simulink model "controllerCoreAlgorithm"  (R2022a)
settings: configuration reference "ControllerCodeGenerationConfigurationSet" (kept outside this file)
model workspace (MATLAB code in the model file + MAT data in the model file):
  cmdLim = Simulink.Parameter
  cmdLim.Value = 15
  cmdLim.Description = 'Limit for controlling the maximum surface command angle.'
  cmdLim.Min = 0
  cmdLim.Max = 90
  cmdLim.DocUnits = 'deg'
  dispGain = Simulink.Parameter
  dispGain.Value = 0.75
  dispGain.Description = 'Gain applied to the displacement error.'
  dispGain.Min = 0
  dispGain.Max = []
  dispGain.DocUnits = 'deg/sec/deg'
  dispLim = Simulink.Parameter
  dispLim.Value = 30
  dispLim.Description = 'Limit for controlling the maximum commanded angle.'
  dispLim.Min = 0
  dispLim.Max = 180
  dispLim.DocUnits = 'deg'
  intGain = Simulink.Parameter
  intGain.Value = 0.5
  intGain.Description = 'Gain applied to the integral error.'
  intGain.Min = 0
  intGain.Max = []
  intGain.DocUnits = 'deg/sec/deg/sec'
  intLim = Simulink.Parameter
  intLim.Value = 5
  intLim.Description = 'Limit for controlling the maximum commanded angle.'
  intLim.Min = 0
  intLim.Max = 90
  intLim.DocUnits = 'deg'
  rateGain = Simulink.Parameter
  rateGain.Value = 2
  rateGain.Description = 'Gain applied to the rate error.'
  rateGain.Min = 0
  rateGain.Max = []
  rateGain.DocUnits = 'deg/deg/sec'
  rateLim = Simulink.Parameter
  rateLim.Value = 6
  rateLim.Description = 'Limit for controlling the maximum commanded angle.'
  rateLim.Min = 0
  rateLim.Max = 180
  rateLim.DocUnits = 'deg/sec'
  hdgGain = Simulink.Parameter
  hdgGain.Value = 0.015
  CLIENT_DEVICE_ID_LIST = Simulink.Parameter
  CLIENT_DEVICE_ID_LIST.Value(1).device_id = [0; 0; 0; 0; 0; 0; 0; 0; 0; 0]
  CLIENT_DEVICE_ID_LIST.Value(2).device_id = [0; 0; 0; 0; 0; 0; 0; 0; 0; 0]
  CLIENT_DEVICE_ID_LIST.Value(3).device_id = [0; 0; 0; 0; 0; 0; 0; 0; 0; 0]
  CLIENT_DEVICE_ID_LIST.Value(4).device_id = [0; 0; 0; 0; 0; 0; 0; 0; 0; 0]
  CLIENT_DEVICE_ID_LIST.Description = 'repmat( SensorTargetSpecificCodeExternalDependency.deviceIDBusTypeDefaultConstructor( ), 4, 1 )'
  CLIENT_DEVICE_ID_LIST.DataType = 'Bus: DeviceIDBusType'
  CLIENT_DEVICE_ID_LIST.Complexity = 'real'
  CLIENT_DEVICE_ID_LIST.Dimensions = [4 1]
  CONTROLLER_SAMPLE_TIME = 0.01
  RECEPTION_LOSS_MESSAGE_INTERVAL = 2
  TIRE_PRESSURE_LOWER_THRESHOLD = 1.4
  TIRE_PRESSURE_UPPER_THRESHOLD = 4.6
undefined symbols (not defined in the file): DEFAULT_DEVICE_ID, DEFAULT_MEASUREMENT_MSG_BUS_TYPE, deviceID, faultCode, FaultCodeEnumType, logFault, PER_STEP_MAXIMUM_MESSAGES_TO_PROCESS
settings Model: RequirementInfo={} %GIDa_fe9045fd_0412_4b6e_8206_617cc20e6fde  DataDictionary=controllerCoreAlgorithmData.sldd  FPTRunName=Active  ParameterArgumentNames=CLIENT_DEVICE_ID_LIST  Creator=The MathWorks, Inc.  LastModifiedBy=The MathWorks, Inc.
settings ConfigSetRef: SourceName=ControllerCodeGenerationConfigurationSet

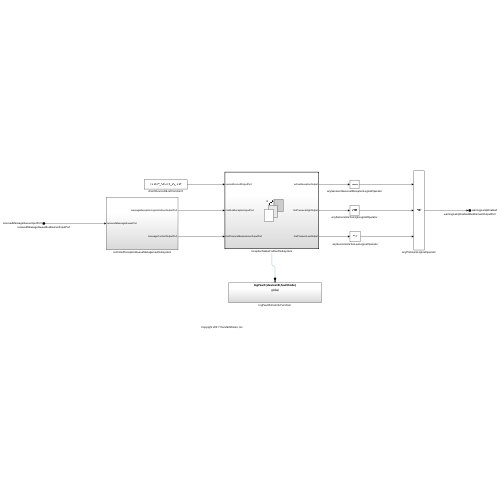
[thumbnail: Simulink's stored preview of the top-level diagram]
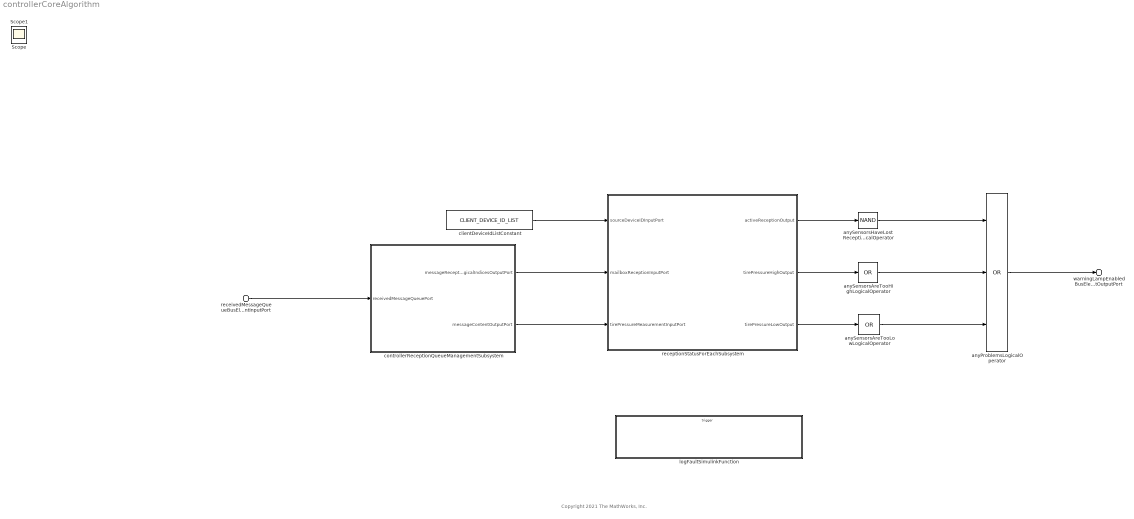
== system controllerCoreAlgorithm ==
  note: Copyright 2021 The MathWorks, Inc.
  receivedMessageQueueBusElementInputPort : Inport  PortName=receivedMessageQueueInputPort
  anyProblemsLogicalOperator : Logic  Operator=OR  Inputs=3  AllPortsSameDT=off  OutDataTypeStr=boolean
  anySensorsAreTooHighLogicalOperator : Logic  Operator=OR  Inputs=1  AllPortsSameDT=off  OutDataTypeStr=boolean
  anySensorsAreTooLowLogicalOperator : Logic  Operator=OR  Inputs=1  AllPortsSameDT=off  OutDataTypeStr=boolean
  anySensorsHaveLostReceptionLogicalOperator : Logic  Operator=NAND  Inputs=1  AllPortsSameDT=off  OutDataTypeStr=boolean
  clientDeviceIdListConstant : Constant  Value=CLIENT_DEVICE_ID_LIST  VectorParams1D=off  OutDataTypeStr=Bus: DeviceIDBusType
  controllerReceptionQueueManagementSubsystem : Subsystem
  logFaultSimulinkFunction : Subsystem  TreatAsAtomicUnit=on
  receptionStatusForEachSubsystem : Subsystem  TreatAsAtomicUnit=on
  warningLampEnabledBusElementOutputPort : Outport  PortName=warningLampEnabled
  Scope : Scope
  Scope1 : Scope
  wires:
  controllerReceptionQueueManagementSubsystem/1(messageReceptionLogicalIndicesOutputPort) -> receptionStatusForEachSubsystem/2(mailboxReceptionInputPort)
  clientDeviceIdListConstant/1 -> receptionStatusForEachSubsystem/1(sourceDeviceIDInputPort)
  receptionStatusForEachSubsystem/1(activeReceptionOutput) -> anySensorsHaveLostReceptionLogicalOperator/1
  receptionStatusForEachSubsystem/2(tirePressureHighOutput) -> anySensorsAreTooHighLogicalOperator/1
  receptionStatusForEachSubsystem/3(tirePressureLowOutput) -> anySensorsAreTooLowLogicalOperator/1
  anySensorsHaveLostReceptionLogicalOperator/1 -> anyProblemsLogicalOperator/1
  anyProblemsLogicalOperator/1 -> warningLampEnabledBusElementOutputPort/1
  anySensorsAreTooHighLogicalOperator/1 -> anyProblemsLogicalOperator/2
  anySensorsAreTooLowLogicalOperator/1 -> anyProblemsLogicalOperator/3
  controllerReceptionQueueManagementSubsystem/2(messageContentOutputPort) -> receptionStatusForEachSubsystem/3(tirePressureMeasurementInputPort)
  receivedMessageQueueBusElementInputPort/1 -> controllerReceptionQueueManagementSubsystem/1(receivedMessageQueuePort)

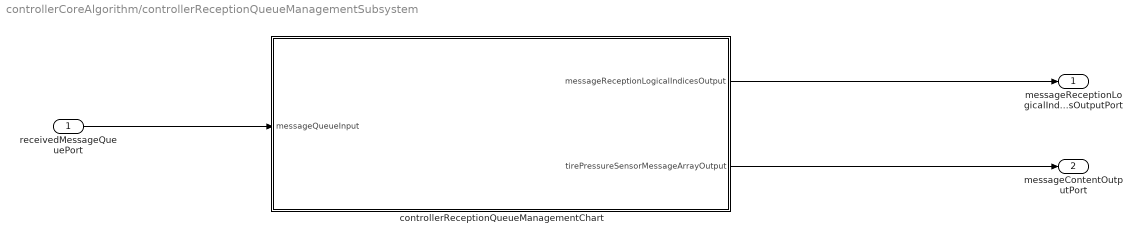
== system controllerCoreAlgorithm/controllerReceptionQueueManagementSubsystem ==
  receivedMessageQueuePort : Inport
  controllerReceptionQueueManagementChart : Stateflow chart  TreatAsAtomicUnit=on
  messageReceptionLogicalIndicesOutputPort : Outport
  messageContentOutputPort : Outport  Port=2
  wires:
  receivedMessageQueuePort/1 -> controllerReceptionQueueManagementChart/1(messageQueueInput)
  controllerReceptionQueueManagementChart/2(tirePressureSensorMessageArrayOutput) -> messageContentOutputPort/1
  controllerReceptionQueueManagementChart/1(messageReceptionLogicalIndicesOutput) -> messageReceptionLogicalIndicesOutputPort/1

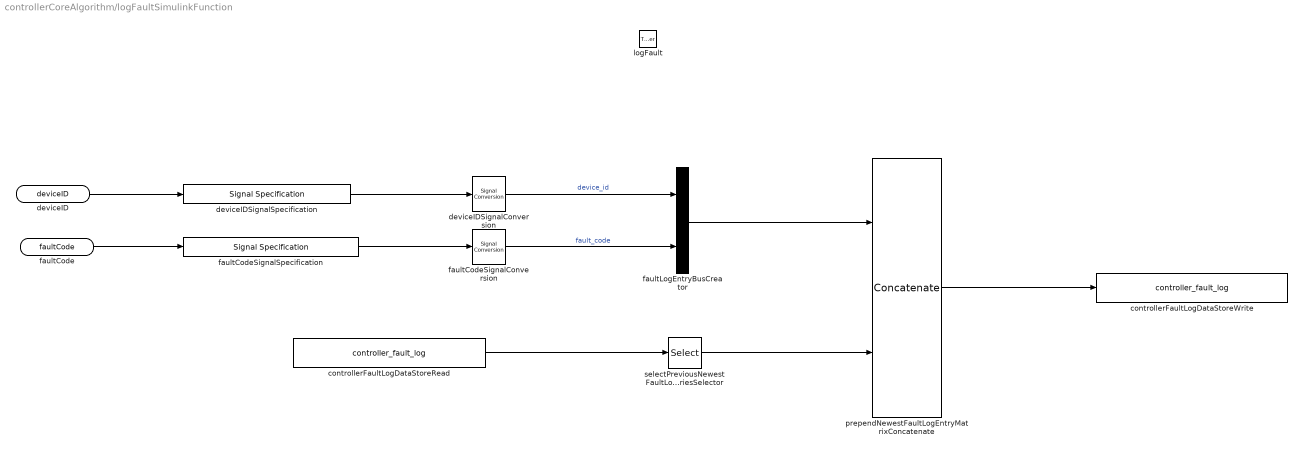
== system controllerCoreAlgorithm/logFaultSimulinkFunction ==
  logFault : TriggerPort  TriggerType=function-call  IsSimulinkFunction=on  FunctionName=logFault  VariantControl=(inherit)
  controllerFaultLogDataStoreRead : DataStoreRead  DataStoreName=controller_fault_log  IndexOptions=Index vector (dialog)  Indices=1  OutputSizes=1
  controllerFaultLogDataStoreWrite : DataStoreWrite  DataStoreName=controller_fault_log  IndexOptions=Index vector (dialog)  Indices=1  OutputSizes=1
  deviceIDSignalConversion : SignalConversion  OverrideOpt=off
  deviceIDSignalSpecification : SignalSpecification  OutDataTypeStr=Bus: DeviceIDBusType  BusOutputAsStruct=on
  faultCodeSignalConversion : SignalConversion  OverrideOpt=off
  faultCodeSignalSpecification : SignalSpecification  OutDataTypeStr=Enum: FaultCodeEnumType
  faultLogEntryBusCreator : BusCreator  Inputs=2  OutDataTypeStr=Bus: ControllerFaultLogEntryBusType  NonVirtualBus=on
  prependNewestFaultLogEntryMatrixConcatenate : Concatenate  Mode=Multidimensional array
  selectPreviousNewestFaultLogEntriesSelector : Selector  InputPortWidth=10  IndexOptions=Index vector (dialog)  Indices=[1: 9]  OutputSizes=1
  deviceID : ArgIn  DisableCoverage=on  OutDataTypeStr=Bus: DeviceIDBusType  ArgumentName=deviceID
  faultCode : ArgIn  DisableCoverage=on  Port=2  OutDataTypeStr=Enum: FaultCodeEnumType  ArgumentName=faultCode
  wires:
  deviceID/1 -> deviceIDSignalSpecification/1
  faultCode/1 -> faultCodeSignalSpecification/1
  deviceIDSignalSpecification/1 -> deviceIDSignalConversion/1
  faultCodeSignalSpecification/1 -> faultCodeSignalConversion/1
  controllerFaultLogDataStoreRead/1 -> selectPreviousNewestFaultLogEntriesSelector/1
  prependNewestFaultLogEntryMatrixConcatenate/1 -> controllerFaultLogDataStoreWrite/1
  faultCodeSignalConversion/1 -> faultLogEntryBusCreator/2  "fault_code"
  deviceIDSignalConversion/1 -> faultLogEntryBusCreator/1  "device_id"
  faultLogEntryBusCreator/1 -> prependNewestFaultLogEntryMatrixConcatenate/1
  selectPreviousNewestFaultLogEntriesSelector/1 -> prependNewestFaultLogEntryMatrixConcatenate/2

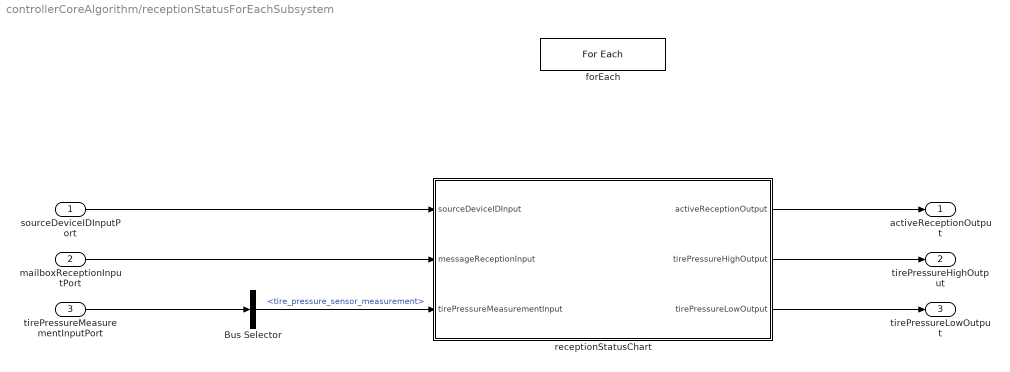
== system controllerCoreAlgorithm/receptionStatusForEachSubsystem ==
  sourceDeviceIDInputPort : Inport  Partition=on  PartitionDimension=1  PartitionWidth=1  PartitionOffset=0
  mailboxReceptionInputPort : Inport  Port=2  Partition=on  PartitionDimension=1  PartitionWidth=1  PartitionOffset=0
  tirePressureMeasurementInputPort : Inport  Port=3  Partition=on  PartitionDimension=1  PartitionWidth=1  PartitionOffset=0
  Bus Selector : BusSelector  OutputSignals=tire_pressure_sensor_measurement
  forEach : ForEach  DisableCoverage=on
  receptionStatusChart : Stateflow chart  TreatAsAtomicUnit=on
      settings: RTWSystemCode=Inline
  activeReceptionOutput : Outport  ConcatenationDimension=1
  tirePressureHighOutput : Outport  Port=2  ConcatenationDimension=1
  tirePressureLowOutput : Outport  Port=3  ConcatenationDimension=1
  wires:
  mailboxReceptionInputPort/1 -> receptionStatusChart/2(messageReceptionInput)
  sourceDeviceIDInputPort/1 -> receptionStatusChart/1(sourceDeviceIDInput)
  receptionStatusChart/1(activeReceptionOutput) -> activeReceptionOutput/1
  receptionStatusChart/2(tirePressureHighOutput) -> tirePressureHighOutput/1
  receptionStatusChart/3(tirePressureLowOutput) -> tirePressureLowOutput/1
  tirePressureMeasurementInputPort/1 -> Bus Selector/1
  Bus Selector/1 -> receptionStatusChart/3(tirePressureMeasurementInput)  "<tire_pressure_sensor_measurement>"

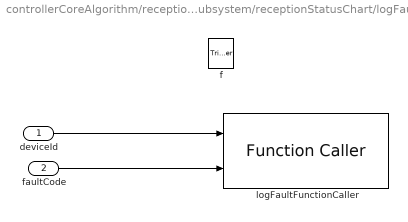
== system controllerCoreAlgorithm/receptionStatusForEachSubsystem/receptionStatusChart/logFaultCallerStateflowSimulinkFunctionWrapper ==
  deviceId : Inport  OutDataTypeStr=Bus: DeviceIDBusType  PortDimensions=1  LockScale=on
  faultCode : Inport  Port=2  OutDataTypeStr=Enum: FaultCodeEnumType  PortDimensions=1
  f : TriggerPort  TriggerType=function-call  VariantControl=(inherit)
      settings: CopyFcn=Stateflow.SLINSF.SimulinkMan.removeBlockPreDeleteFcn  PreDeleteFcn=Stateflow.SLINSF.SimulinkMan.unsafePredeleteFcn
  logFaultFunctionCaller : FunctionCaller  FunctionPrototype=logFault(deviceID,faultCode)  InputArgumentSpecifications=DEFAULT_DEVICE_ID, FaultCodeEnumType.getDefaultValue( )  OutputArgumentSpecifications=<Enter example>
  wires:
  deviceId/1 -> logFaultFunctionCaller/1
  faultCode/1 -> logFaultFunctionCaller/2

== stateflow chart controllerCoreAlgorithm/receptionStatusForEachSubsystem/receptionStatusChart ==
  state logFaultCallerStateflowSimulinkFunctionWrapper( deviceId, faultCode ) [function]
  state RECEPTION_LOST
    entry:
    activeReceptionOutput = false;
  state WAITING_FOR_RECEPTION
    entry:
    activeReceptionOutput = true;
  (default) -> WAITING_FOR_RECEPTION : {
      | activeReceptionOutput = true;
      | tirePressureHighOutput = false;
      | tirePressureLowOutput = false;
      | }
  WAITING_FOR_RECEPTION -> RECEPTION_LOST [order 2] : [ after( RECEPTION_LOSS_MESSAGE_INTERVAL, sec ) ]
      | {
      | logFaultCallerStateflowSimulinkFunctionWrapper( sourceDeviceIDInput, FaultCodeEnumType.RECEPTION_LOSS_FAULT_CODE_EN );
      | }
  (junction 40) -> WAITING_FOR_RECEPTION
  WAITING_FOR_RECEPTION -> (junction 59) [order 1] : [ true == messageReceptionInput ]
  RECEPTION_LOST -> (junction 59) : [ true == messageReceptionInput ]
  (junction 59) -> (junction 16)
  (junction 16) -> (junction 17) [order 1] : [ tirePressureMeasurementInput > TIRE_PRESSURE_UPPER_THRESHOLD ]
  (junction 16) -> (junction 44) [order 2] : {
      | tirePressureHighOutput = false;
      | }
  (junction 17) -> (junction 45) : {
      | tirePressureHighOutput = true;
      | logFaultCallerStateflowSimulinkFunctionWrapper( sourceDeviceIDInput, FaultCodeEnumType.HIGH_PRESSURE_FAULT_CODE_EN );
      | }
  (junction 45) -> (junction 44)
  (junction 44) -> (junction 32)
  (junction 32) -> (junction 34) [order 1] : [ tirePressureMeasurementInput < TIRE_PRESSURE_LOWER_THRESHOLD ]
  (junction 32) -> (junction 37) [order 2] : {
      | tirePressureLowOutput = false;
      | }
  (junction 34) -> (junction 30) : {
      | tirePressureLowOutput = true;
      | logFaultCallerStateflowSimulinkFunctionWrapper( sourceDeviceIDInput, FaultCodeEnumType.LOW_PRESSURE_FAULT_CODE_EN );
      | }
  (junction 37) -> (junction 40)
  (junction 30) -> (junction 37)
  data: deviceId function_input Bus: DeviceIDBusType size=1; faultCode function_input Enum: FaultCodeEnumType size=1; sourceDeviceIDInput input Bus: DeviceIDBusType; messageReceptionInput input; TIRE_PRESSURE_UPPER_THRESHOLD parameter; TIRE_PRESSURE_LOWER_THRESHOLD parameter; tirePressureMeasurementInput input; activeReceptionOutput output; tirePressureHighOutput output; tirePressureLowOutput output; RECEPTION_LOSS_MESSAGE_INTERVAL parameter

== stateflow chart controllerCoreAlgorithm/controllerReceptionQueueManagementSubsystem/controllerReceptionQueueManagementChart ==
  (default) -> (junction 63) : {
      |
      | localProcessedMessageCount = uint8( 1 );
      |
      | messageReceptionLogicalIndicesOutput = ...
      |     false( size( CLIENT_DEVICE_ID_LIST ) );
      |
      | tirePressureSensorMessageArrayOutput = ...
      |     repmat( DEFAULT_MEASUREMENT_MSG_BUS_TYPE, size( CLIENT_DEVICE_ID_LIST ) );
      | }
  (junction 63) -> (junction 69) [order 2] : % Per-step message processing limit exceeded.
  (junction 66) -> (junction 63)
  (junction 63) -> (junction 2) [order 1] : [ localProcessedMessageCount < PER_STEP_MAXIMUM_MESSAGES_TO_PROCESS ]
  (junction 50) -> (junction 66)
  (junction 69) -> (junction 13)
  (junction 2) -> (junction 13) [order 2] : % There are no messages.
  (junction 2) -> (junction 50) [order 1] : [ receive( messageQueueInput ) ]
      | {
      |
      | [ tirePressureSensorMessageArrayOutput, messageReceptionLogicalIndicesOutput ] = ...
      |     insert_message_in_mailbox( tirePressureSensorMessageArrayOutput, messageReceptionLogicalIndicesOutput, messageQueueInput.data, CLIENT_DEVICE_ID_LIST );
      | discard( messageQueueInput );
      | localProcessedMessageCount = localProcessedMessageCount + 1;
      |
      | }
  (junction 13) -> (junction 55) : % Done.
  data: originalMailboxes function_input; originalMailboxFlags function_input; candidateMessage function_input; mailboxDeviceIDList function_input; updatedMailboxes function_output; updatedMailboxFlags function_output; CLIENT_DEVICE_ID_LIST parameter; messageReceptionLogicalIndicesOutput output; tirePressureSensorMessageArrayOutput output Bus: MeasurementMsgBusType; messageQueueInput input; DEFAULT_MEASUREMENT_MSG_BUS_TYPE parameter; localProcessedMessageCount local; PER_STEP_MAXIMUM_MESSAGES_TO_PROCESS parameter uint8
  function [ updatedMailboxes, updatedMailboxFlags ] = insert_message_in_mailbox( originalMailboxes, originalMailboxFlags, candidateMessage, mailboxDeviceIDList ):
    | function [ updatedMailboxes, updatedMailboxFlags ] = insert_message_in_mailbox( originalMailboxes, originalMailboxFlags, candidateMessage, mailboxDeviceIDList )
    | 
    | assert( numel( mailboxDeviceIDList) == numel( originalMailboxes) );
    | 
    | updatedMailboxFlags = originalMailboxFlags;
    | updatedMailboxes = originalMailboxes;
    | 
    | currentCandidateMessageDeviceID = candidateMessage.source.device_id;
    | 
    | clientDeviceQuantity = uint8( numel( mailboxDeviceIDList) );
    | 
    | for messageIDSearchIndex = 1 : clientDeviceQuantity
    | 
    |     % The "device_id" field is an array of integers, so "all" is necessary
    |     % to check all elements of this list.
    |     currentMailboxDeviceID = mailboxDeviceIDList( messageIDSearchIndex ).device_id;
    |     
    |     if( true == all( currentMailboxDeviceID == currentCandidateMessageDeviceID ) )
    |         updatedMailboxFlags( messageIDSearchIndex ) = true;
    |         updatedMailboxes( messageIDSearchIndex) = candidateMessage;
    |         break;
    |     else
    |         % Keep searching.
    |     end
    | end
    | 
    | return;
    | 
    | end
